simulink model "pd_ctrl"  (R2020b)
settings: Solver=VariableStepAuto  StartTime=0.0  StopTime=10.0  RelTol=1e-3
values from neighbouring files (symbols this model uses):
  Kd = 2*zeta*wn    (= 10)    [script_pd.m]
  Kp = wn^2    (= 25)    [script_pd.m]
  q0 = [0 0 0 0]'    [script_pd.m]
undefined symbols (not defined in the file or in its folder): traj_switch
settings Model: Creator=lucas  LastModifiedBy=lucas

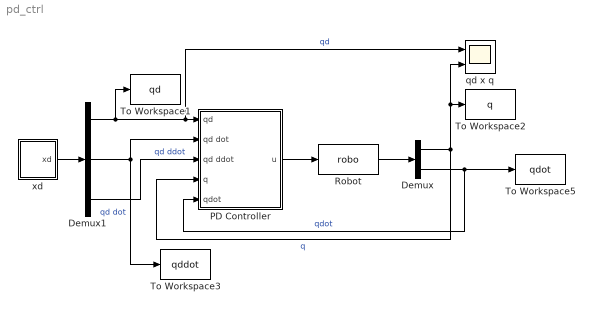
== system pd_ctrl ==
  Demux : Demux  Outputs=2
  Demux1 : Demux  Outputs=3
  PD Controller : Subsystem
  Robot : S-Function  FunctionName=robo  Parameters=q0  SFunctionDeploymentMode=off  EnableBusSupport=off  mask(Robot){xi=q0}
      mask prompts: xi "Condicao Inicial"
  To Workspace1 : ToWorkspace  VariableName=qd  SaveFormat=Timeseries  SampleTime=-1
  To Workspace2 : ToWorkspace  VariableName=q  SaveFormat=Timeseries  SampleTime=-1
  To Workspace3 : ToWorkspace  VariableName=qddot  SaveFormat=Timeseries  SampleTime=-1
  To Workspace5 : ToWorkspace  VariableName=qdot  SaveFormat=Timeseries  SampleTime=-1
  qd x q : Scope  NumInputPorts=2
  xd : Subsystem
  wires:
  xd/1(xd) -> Demux1/1
  Robot/1 -> Demux/1
  Demux1/1 -> To Workspace1/1, qd x q/1, PD Controller/1(qd)  "qd"
  Demux/1 -> qd x q/2, To Workspace2/1, PD Controller/4(q)  "q"
  Demux1/2 -> To Workspace3/1, PD Controller/2(qd dot)  "qd dot"
  Demux/2 -> PD Controller/5(qdot), To Workspace5/1  "qdot"
  Demux1/3 -> PD Controller/3(qd ddot)  "qd ddot"
  PD Controller/1(u) -> Robot/1

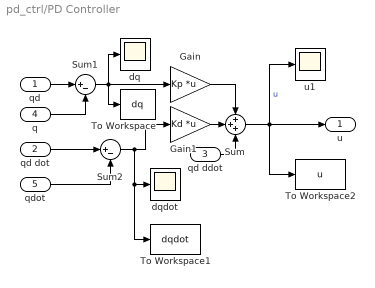
== system pd_ctrl/PD Controller ==
  qd : Inport
  qd dot : Inport  Port=2
  qd ddot : Inport  Port=3
  q : Inport  Port=4
  qdot : Inport  Port=5
  Gain : Gain  Gain=Kp  Multiplication=Matrix(K*u)
  Gain1 : Gain  Gain=Kd  Multiplication=Matrix(K*u)
  Sum : Sum  Inputs=+++
  Sum1 : Sum  Inputs=|+-
  Sum2 : Sum  Inputs=|+-
  To Workspace : ToWorkspace  VariableName=dq  SaveFormat=Timeseries  SampleTime=-1
  To Workspace1 : ToWorkspace  VariableName=dqdot  SaveFormat=Timeseries  SampleTime=-1
  To Workspace2 : ToWorkspace  VariableName=u  SaveFormat=Timeseries  SampleTime=-1
  dq : Scope
  dqdot : Scope
  u1 : Scope
  u : Outport
  wires:
  qd dot/1 -> Sum2/1
  Sum/1 -> u/1, u1/1, To Workspace2/1  "u"
  qd/1 -> Sum1/1
  Gain/1 -> Sum/1
  Sum2/1 -> To Workspace1/1, dqdot/1, Gain1/1
  Sum1/1 -> dq/1, To Workspace/1, Gain/1
  qdot/1 -> Sum2/2
  Gain1/1 -> Sum/2
  qd ddot/1 -> Sum/3
  q/1 -> Sum1/2

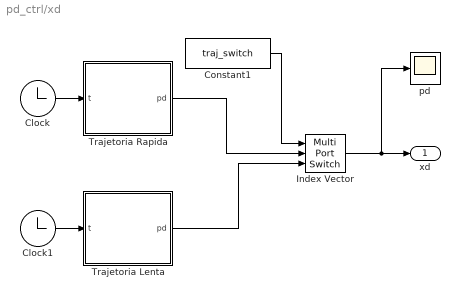
== system pd_ctrl/xd ==
  Clock : Clock
  Clock1 : Clock
  Constant1 : Constant  Value=traj_switch
  Index Vector : MultiPortSwitch  DataPortOrder=Zero-based contiguous  Inputs=2  zeroidx=on
  Trajetoria Lenta : MATLAB Function  TreatAsAtomicUnit=on
  Trajetoria Rapida : MATLAB Function  TreatAsAtomicUnit=on
  pd : Scope
  xd : Outport
  wires:
  Trajetoria Lenta/1(pd) -> Index Vector/3
  Clock/1 -> Trajetoria Rapida/1(t)
  Constant1/1 -> Index Vector/1
  Trajetoria Rapida/1(pd) -> Index Vector/2
  Clock1/1 -> Trajetoria Lenta/1(t)
  Index Vector/1 -> pd/1, xd/1

== matlab function pd_ctrl/xd/Trajetoria Lenta ==
  data: pd output; t input
function pd = fcn(t)
qd = [(-0.75*cos(pi*t/2))-0.75; (-0.75*cos(pi*t/2))+3.75];

qddot = [0.75*(pi/2)*sin(pi*t/2); 0.75*(pi/2)*sin(pi*t/2)];

qdddot = [0.75*(pi/2)^2*cos(pi*t/2); 0.75*(pi/2)^2*cos(pi*t/2)];

pd = [qd;qddot;qdddot];

== matlab function pd_ctrl/xd/Trajetoria Rapida ==
  data: pd output; t input
function pd = fcn(t)
qd = [(-0.75*cos(pi*t))-0.75; (-0.75*cos(pi*t))+3.75];

qddot = [0.75*pi*sin(pi*t); 0.75*pi*sin(pi*t)];

qdddot = [0.75*pi^2*cos(pi*t); 0.75*pi^2*cos(pi*t)];

pd = [qd;qddot;qdddot];
